simulink model "OFDM2017a"  (R2017a)
settings: Solver=FixedStepDiscrete  StartTime=0.0  StopTime=inf  RelTol=1e-3
PreLoadFcn:
  | nbZeros = 12
  | nbPilots = 4
  | signalSize = 16
InitFcn:
  | nbZeros = 12
  | nbPilots = 4
  | signalSize = 16
libraries: dspxfrm3 x2, commdigbbndpm3 x2, commrandsrc3 x1, commsink2 x1, commchan3 x1
settings Model: SimulationMode=accelerator  Creator=pchabance  LastModifiedBy=Antoine
settings SolverCC: AutoInsertRateTranBlk=on
settings DataIOCC: LimitDataPoints=on  SaveOutput=off  SignalLogging=off  SaveTime=off
settings OptimizationCC: LifeSpan=inf
settings DebuggingCC: AlgebraicLoopMsg=error  SingleTaskRateTransMsg=error  AllowSymbolicDim=off  SFUnexpectedBacktrackingDiag=warning  SFNoUnconditionalDefaultTransitionDiag=warning  SFExecutionAtInitializationDiag=none
settings GRTTargetCC: TargetLangStandard=C89/C90 (ANSI)  GeneratePreprocessorConditionals=Disable all

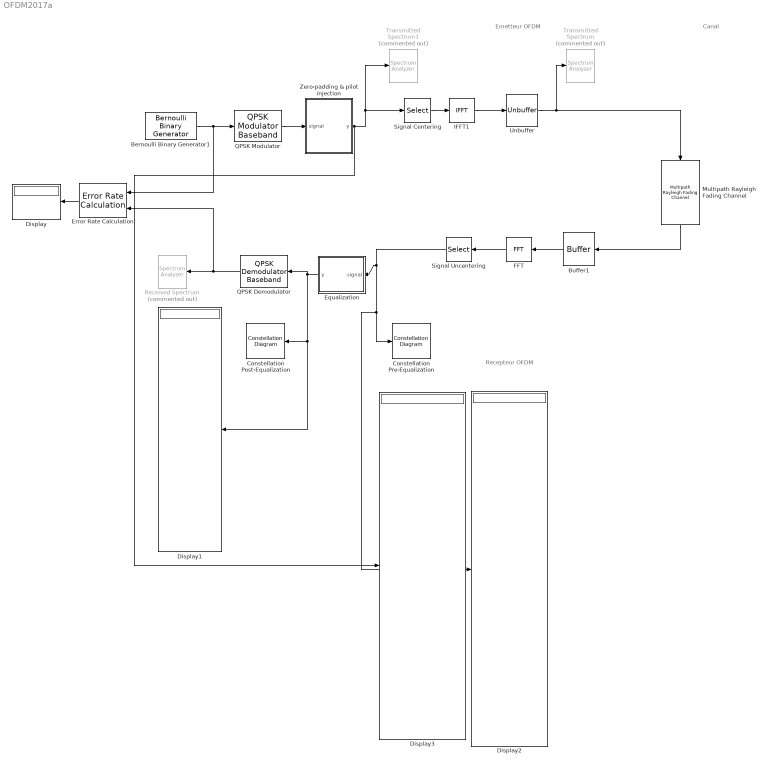
== system OFDM2017a ==
  note: Emetteur OFDM
  note: Recepteur OFDM
  note: Canal
  Bernoulli Binary Generator1 : commrandsrc3/Bernoulli Binary Generator  ProbabilityOfZero=0.5  SeedSource=Auto  Seed=0  SampleTime=1e-6/32  SamplesPerFrame=32  OutputDataType=double  SimulateUsing=Code generation
      settings: SourceProductName=Communications Toolbox
  Buffer1 : Buffer  N=32  OutputFrames=off
  Constellation Post-Equalization : ConstellationDiagram
  Constellation Pre-Equalization : ConstellationDiagram
  Display{,1..3} (4 alike) : Display
  Equalization : MATLAB Function  TreatAsAtomicUnit=on
  Error Rate Calculation : commsink2/Error Rate Calculation  N=32  st_delay=0  cp_mode=Entire frame  subframe=[]  PMode=Port  WsName=ErrorVec  RsMode2=off  stop=off  numErr=100  maxBits=1e6
      settings: SourceProductName=Communications Toolbox
  FFT : dspxfrm3/FFT  FFTImplementation=Auto  CompMethod=Table lookup  TableOpt=NEW  TableOptActive=Speed  BitRevOrder=off  Normalize=off  InheritFFTLength=on  FFTLength=64  WrapInput=on  roundingMode=Floor  overflowMode=off  firstCoeffDataTypeStr=Inherit: Same word length as input  firstCoeffLastDataTypeStr=Inherit: Same word length as input  outputMin=[]  outputMax=[]
  IFFT1 : dspxfrm3/IFFT  FFTImplementation=Auto  CompMethod=Table lookup  TableOpt=NEW  TableOptActive=Speed  BitRevOrder=off  cs_in=off  Normalize=on  InheritFFTLength=on  FFTLength=64  WrapInput=on  mode=Complex  outSamplingMode=Sample based  roundingMode=Floor  overflowMode=off  firstCoeffDataTypeStr=Inherit: Same word length as input  firstCoeffLastDataTypeStr=Inherit: Same word length as input  outputMin=[]  outputMax=[]
      settings: SourceProductName=DSP System Toolbox
  Multipath Rayleigh Fading Channel : commchan3/Multipath Rayleigh Fading Channel  maxDopplerShift=40  spectrumType=Specify as dialog parameter  sigmaGaussian=[]  coeffRounded=[]  freqMinMaxRJakes=[]  freqMinMaxAJakes=[]  sigmaGaussian1=[]  sigmaGaussian2=[]  centerFreqGaussian1=[]  centerFreqGaussian2=[]  gainGaussian1=[]  gainGaussian2=[]  coeffBell=[]  dopplerSpectrum=doppler.jakes  pathDelays=[0 0]  avgPathGaindB=[0 -3]  normalizePathGains=on  seed=73  enableProbe=0  openVisAtStart=off  outPathGains=off  outDelay=off
  "QPSK Demodulator " : commdigbbndpm3/QPSK Demodulator Baseband  OutType=Bit  DecType=Hard decision  VarSource=Dialog  Variance=1  Dec=Gray  Ph=pi/4  outDtype1=Inherit via internal rule  outDtype2=Inherit via internal rule  derotateFactorWordLen=16  derotateFactorDataTypeStr=Inherit: Same word length as input  derotateFactorLastDataTypeStr=Inherit: Same word length as input
      settings: SourceProductName=Communications Toolbox
  "QPSK Modulator " : commdigbbndpm3/QPSK Modulator Baseband  InType=Bit  Enc=Gray  Ph=pi/4  outDtype=double  outWordLen=16  outUDDataType=sfix(16)  outFracLenMode=Best precision  outFracLen=15  outDataTypeStr=double  outLastDataTypeStr=double
      settings: SourceProductName=Communications Toolbox
  Received Spectrum : SpectrumAnalyzer  Commented=on
  Signal Uncentering : Selector  InputPortWidth=32  IndexOptions=Index vector (dialog)  Indices=[18:32 1:17]  OutputSizes=1
  Signal Centering : Selector  InputPortWidth=32  IndexOptions=Index vector (dialog)  Indices=[16:32 1:15]  OutputSizes=1
  Transmitted Spectrum : SpectrumAnalyzer  Commented=on
  Transmitted Spectrum1 : SpectrumAnalyzer  Commented=on
  Unbuffer : Unbuffer
  Zero-padding & pilot injection : MATLAB Function  TreatAsAtomicUnit=on
  wires:
  "QPSK Modulator "/1 -> Zero-padding & pilot injection/1(signal)
  Signal Centering/1 -> IFFT1/1
  IFFT1/1 -> Unbuffer/1
  Unbuffer/1 -> Multipath Rayleigh Fading Channel/1, Transmitted Spectrum/1
  Buffer1/1 -> FFT/1
  FFT/1 -> Signal Uncentering/1
  "QPSK Demodulator "/1 -> Error Rate Calculation/2, Received Spectrum/1
  Error Rate Calculation/1 -> Display/1
  Bernoulli Binary Generator1/1 -> Error Rate Calculation/1, "QPSK Modulator "/1
  Multipath Rayleigh Fading Channel/1 -> Buffer1/1
  Signal Uncentering/1 -> Constellation Pre-Equalization/1, Display2/1, Equalization/1(signal)
  Equalization/1(y) -> "QPSK Demodulator "/1, Constellation Post-Equalization/1, Display1/1
  Zero-padding & pilot injection/1(y) -> Display3/1, Transmitted Spectrum1/1, Signal Centering/1

== matlab function OFDM2017a/Equalization ==
  data: y output size=[signalSize,1]; signal input; nbPilots parameter; signalSize parameter; nbZeros parameter
function y = fcn(signal, nbPilots, signalSize, nbZeros)

    signalSansZeros = signal(nbZeros/2+1:nbZeros/2+signalSize+nbPilots);

    intervalle = floor(signalSize/nbPilots)+1;
    output = zeros(signalSize,1) + 1j * zeros(signalSize,1);
    indexOutput = 1;
    
    coeffs = zeros(nbPilots,1)+ 1j*zeros(nbPilots,1);
    indexCoeffs = 1;
    
    for i = 1:signalSize+nbPilots
        if mod(i+floor(intervalle/2),intervalle) == 0
            disp('index pilot  :')
            i
            coeffs(indexCoeffs) = (3+3j)/signalSansZeros(i);
            indexCoeffs = indexCoeffs + 1;
        end
    end
    
    indexCoeffs = 1;
    
    for i = 1:signalSize+nbPilots
        if mod(i+floor(intervalle/2),intervalle) ~= 0
            output(indexOutput) = signalSansZeros(i)*coeffs(indexCoeffs);
            indexOutput = indexOutput + 1;
        end
        if mod(i,2*intervalle+1) == 0
            indexCoeffs = indexCoeffs + 1;
        end
    end

y = output;

== matlab function OFDM2017a/Zero-padding & pilot injection ==
  data: y output size=[nbZeros+nbPilots+signalSize,1]; nbZeros parameter; nbPilots parameter; signal input size=16; signalSize parameter
function y = fcn(nbZeros, nbPilots, signal, signalSize)

    index = 1;
    
    intervalle = floor(signalSize/nbPilots)+1;
    output = zeros(nbZeros+nbPilots+signalSize,1)+1j * zeros(nbZeros+nbPilots+signalSize,1);
    
    for i=nbZeros/2+1:signalSize+nbZeros/2+nbPilots
        if mod(i-nbZeros/2+floor(intervalle/2),intervalle) == 0
            output(i)= 3+3j;
        else
            output(i)=signal(index);
            index = index+1;
        end
    end
y = output;
